simulink model "SegOrdem"  (R2015a)
settings: Solver=ode45  StartTime=0.0  StopTime=200  FixedStep=0.00001  RelTol=1e-5
settings Model: Creator=user  LastModifiedBy=user
settings SolverCC: ZeroCrossAlgorithm=Adaptive
settings DebuggingCC: UnderspecifiedInitializationDetection=Classic

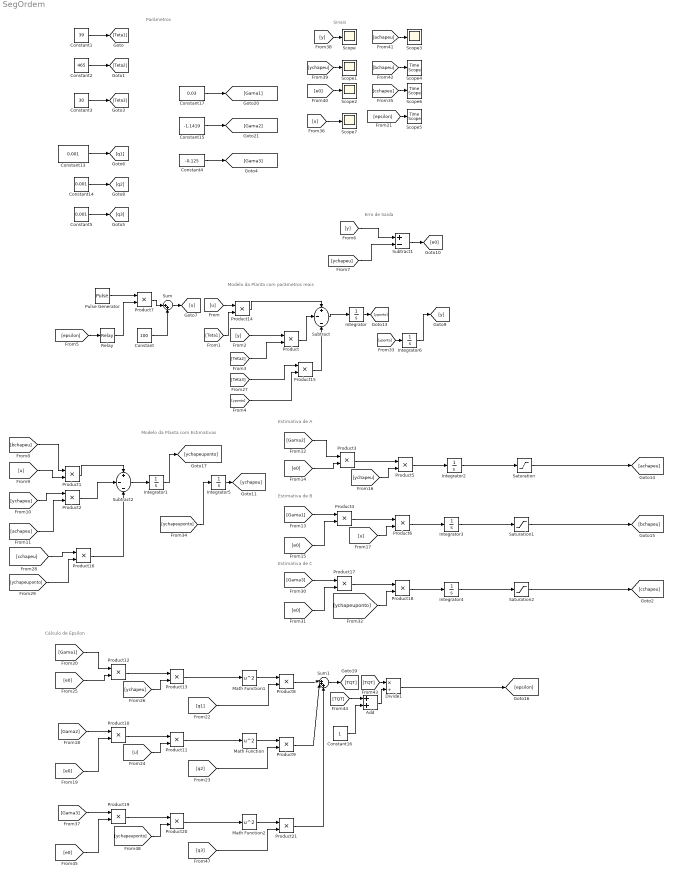
== system SegOrdem ==
  note: Cálculo de Epsilon
  note: Estimativa de B
  note: Estimativa de A
  note: Modelo da Planta com Estimativas
  note: Modelo da Planta com parâmetros reais
  note: Erro de Saída
  note: Parâmetros
  note: Sinais
  note: Estimativa de C
  Add : Sum  AccumDataTypeStr=double
  Constant : Constant  Value=100
  Constant1 : Constant  Value=39
  Constant13 : Constant  Value=0.001
  Constant14 : Constant  Value=0.001
  Constant15 : Constant  Value=-1.1419
  Constant16 : Constant
  Constant17 : Constant  Value=0.03
  Constant2 : Constant  Value=465
  Constant3 : Constant  Value=30
  Constant4 : Constant  Value=-0.125
  Constant5 : Constant  Value=0.001
  Divide1 : Product  Inputs=*/  OutDataTypeStr=double
  Integrator{,1,5..6} (4 alike) : Integrator
  Integrator2 : Integrator  InitialCondition=70
  Integrator3 : Integrator  InitialCondition=80
  Integrator4 : Integrator  InitialCondition=5
  Math Function : Math  Operator=square  SaturateOnIntegerOverflow=on
  Math Function1 : Math  Operator=square  SaturateOnIntegerOverflow=on
  Math Function2 : Math  Operator=square  SaturateOnIntegerOverflow=on
  Product{,1..21} (22 alike) : Product
  Pulse Generator : DiscretePulseGenerator  PulseType=Time based  Amplitude=100  Period=0.1  PulseWidth=50
  Relay : Relay  OnSwitchValue=0.5  OffSwitchValue=0.5
  Saturation : Saturate  UpperLimit=50000  LowerLimit=0
  Saturation1 : Saturate  UpperLimit=300000  LowerLimit=1
  Saturation2 : Saturate  UpperLimit=30000  LowerLimit=0
  Scope{,1..3,7} (5 alike) : Scope
      Scope settings: YMin=11.75  YMax=12.6
      Scope1 settings: YMin=0  YMax=27.5  SampleInput=on
      Scope2 settings: YMin=-12  YMax=12  SaveName=ScopeData2  SampleInput=on
      Scope3 settings: YMin=476  YMax=478.75  SaveName=ScopeData3  SampleInput=on
      Scope7 settings: YMin=-12  YMax=12  SaveName=ScopeData5  SampleInput=on
  Scope4 : TimeScope
  Scope5 : TimeScope
  Scope6 : TimeScope
  Subtract : Sum  Inputs=+--
  Subtract1 : Sum  Inputs=+-
  Subtract2 : Sum  Inputs=+--
  Sum : Sum  Inputs=|++
  Sum1 : Sum  Inputs=|+++
  wires:
  Constant/1 -> Sum/2
  [Teta1] -> Product14/2
  [Teta2] -> Product/2
  Product/1 -> Subtract/2
  Product14/1 -> Subtract/1
  Subtract/1 -> Integrator/1
  [y] -> Product/1
  Sum/1 -> [u]
  [u] -> Product14/1
  [y] -> Subtract1/1
  [ychapeu] -> Subtract1/2
  Subtract1/1 -> [e0]
  Constant1/1 -> [Teta1]
  Constant2/1 -> [Teta2]
  Product1/1 -> Subtract2/1
  Subtract2/1 -> Integrator1/1
  Product2/1 -> Subtract2/2
  [achapeu] -> Product2/2
  [ychapeu] -> Product2/1
  [u] -> Product1/2
  [bchapeu] -> Product1/1
  [e0] -> Product3/2
  [Gama2] -> Product3/1
  [Gama1] -> Product4/1
  [e0] -> Product4/2
  Product4/1 -> Product6/1
  Product3/1 -> Product5/1
  [ychapeu] -> Product5/2
  [u] -> Product6/2
  Product5/1 -> Integrator2/1
  Product6/1 -> Integrator3/1
  Integrator3/1 -> Saturation1/1
  Integrator2/1 -> Saturation/1
  Product7/1 -> Sum/1
  Pulse Generator/1 -> Product7/1
  Product11/1 -> Math Function/1
  Product13/1 -> Math Function1/1
  Math Function1/1 -> Product8/1
  Math Function/1 -> Product9/1
  [q1] -> Product8/2
  [q2] -> Product9/2
  Product9/1 -> Sum1/2
  Product8/1 -> Sum1/1
  Constant13/1 -> [q1]
  Constant14/1 -> [q2]
  [y] -> Scope/1
  [ychapeu] -> Scope1/1
  [e0] -> Scope2/1
  [achapeu] -> Scope3/1
  [bchapeu] -> Scope4/1
  Constant17/1 -> [Gama1]
  Constant15/1 -> [Gama2]
  Add/1 -> Divide1/2
  Constant16/1 -> Add/2
  Sum1/1 -> [TQT]
  [TQT] -> Divide1/1
  [TQT] -> Add/1
  [epsilon] -> Relay/1
  Saturation/1 -> [achapeu]
  Saturation1/1 -> [bchapeu]
  [Gama2] -> Product10/1
  [e0] -> Product10/2
  Product10/1 -> Product11/1
  [u] -> Product11/2
  [e0] -> Product12/2
  [Gama1] -> Product12/1
  Product12/1 -> Product13/1
  [ychapeu] -> Product13/2
  Relay/1 -> Product7/2
  [epsilon] -> Scope5/1
  [yponto] -> Product15/2
  [Teta3] -> Product15/1
  Product15/1 -> Subtract/3
  [ychapeuponto] -> Product16/2
  [cchapeu] -> Product16/1
  Product16/1 -> Subtract2/3
  [Gama3] -> Product17/1
  [e0] -> Product17/2
  Product17/1 -> Product18/1
  [ychapeuponto] -> Product18/2
  Product18/1 -> Integrator4/1
  Integrator4/1 -> Saturation2/1
  Saturation2/1 -> [cchapeu]
  Constant3/1 -> [Teta3]
  Constant4/1 -> [Gama3]
  Constant5/1 -> [q3]
  Integrator5/1 -> [ychapeu]
  Integrator6/1 -> [y]
  Integrator/1 -> [yponto]
  [yponto] -> Integrator6/1
  [ychapeuponto] -> Integrator5/1
  Integrator1/1 -> [ychapeuponto]
  [cchapeu] -> Scope6/1
  Divide1/1 -> [epsilon]
  [u] -> Scope7/1
  Product20/1 -> Math Function2/1
  Math Function2/1 -> Product21/1
  [q3] -> Product21/2
  [Gama3] -> Product19/1
  [e0] -> Product19/2
  Product19/1 -> Product20/1
  [ychapeuponto] -> Product20/2
  Product21/1 -> Sum1/3
